simulink model "RL_Check"  (R2020a)
settings: Solver=FixedStepAuto  StartTime=0.0  StopTime=10.0  FixedStep=1e-4  RelTol=1e-3
libraries: commchan3 x1
settings Model: Creator=niranjan.bhujel  LastModifiedBy=niranjan.bhujel

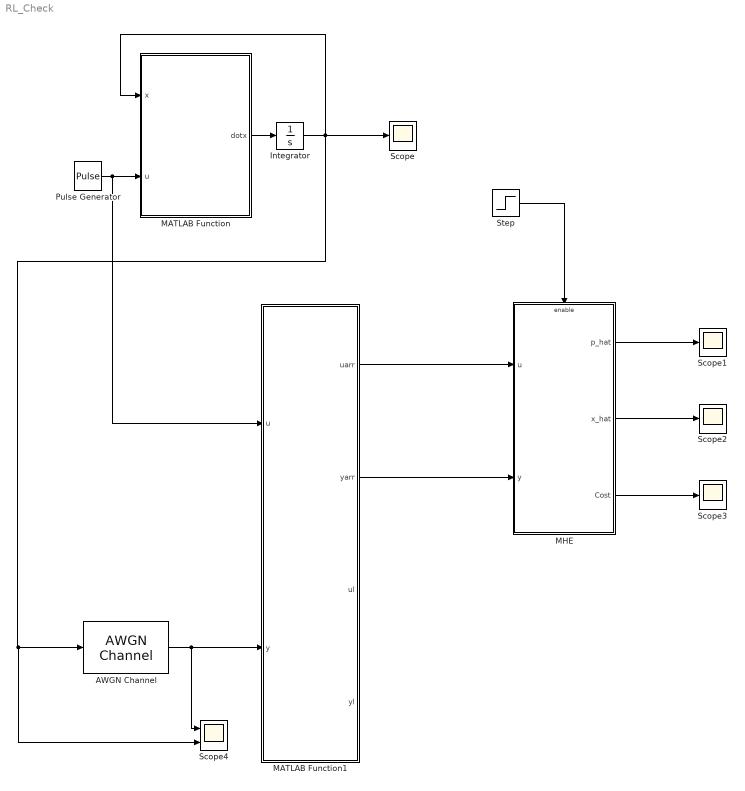
== system RL_Check ==
  AWGN Channel : commchan3/AWGN Channel  InputProcessing=Columns as channels (frame based)  seed=67  noiseMode=Variance from mask  EbNodB=10  EsNodB=10  SNRdB=10  bitsPerSym=1  Ps=1  Tsym=1  variance=1e-3
  Integrator : Integrator
  MATLAB Function : MATLAB Function  TreatAsAtomicUnit=on
  MATLAB Function1 : MATLAB Function  TreatAsAtomicUnit=on  SystemSampleTime=0.005
  MHE : Subsystem
  Pulse Generator : DiscretePulseGenerator  PulseType=Time based  Period=0.5  PulseWidth=50
  Scope{,1..3} (4 alike) : Scope
  Scope4 : Scope  NumInputPorts=2
  Step : Step  Time=5  SampleTime=0
  wires:
  MATLAB Function/1(dotx) -> Integrator/1
  Integrator/1 -> Scope4/2, AWGN Channel/1, Scope/1, MATLAB Function/1(x)
  Pulse Generator/1 -> MATLAB Function1/1(u), MATLAB Function/2(u)
  MATLAB Function1/1(uarr) -> MHE/1(u)
  MATLAB Function1/2(yarr) -> MHE/2(y)
  MHE/1(p_hat) -> Scope1/1
  MHE/2(x_hat) -> Scope2/1
  MHE/3(Cost) -> Scope3/1
  Step/1 -> MHE/Enable
  AWGN Channel/1 -> Scope4/1, MATLAB Function1/2(y)

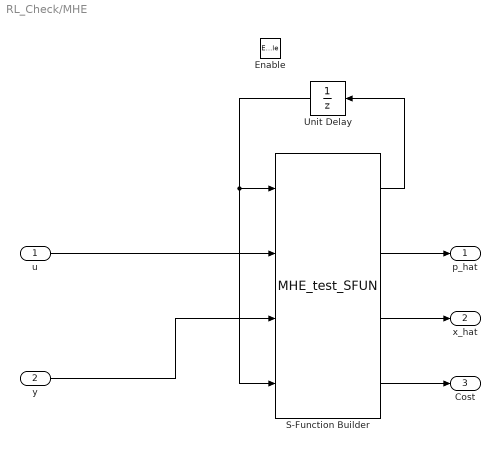
== system RL_Check/MHE ==
  u : Inport
  y : Inport  Port=2
  Enable : EnablePort
  S-Function Builder : S-Function  InitFcn=try, set_param(gcb,'FunctionName','MHE_test_SFUN'), end  FunctionName=MHE_test_SFUN  SFunctionModules=MHE_test_SFUN_wrapper MHE_Code MHE_Code_Call  SFunctionDeploymentMode=off  EnableBusSupport=off  mask(S-Function Builder){}
      mask help: Simulink:masks:SFunctionBuilder_MD
      mask init:
      | val = [[.9  0.75 0.75 1 1 .9 .9 1]',[1 1 0.75 0.75 .9 .9 1 .9]'];try , sys = get_param(gcb,'SfunBuilderFcnName');if isempty(sys), sys = get_param(gcb,'FunctionName'); end,catch, sys = get_param(gcb,'FunctionName'); end
      settings: CopyFcn=set_param(gcbh,'LinkStatus','none')  PreSaveFcn=try, set_param(gcb,'FunctionName','MHE_test_SFUN'), end  OpenFcn=sfunctionwizard(gcbh)
      mask Display: plot(val(:,1),val(:,2)),disp(sys), port_label('input',1,'zGuess'), port_label('input',2,'um'), port_label('input',3,'ym'), port_label('input',4,'zOp'), port_label('output',1,'zOut'), port_label('output',2,'p_hat'), port_label('output',3,'x_hat'), port_label('output',4,'Cost')
  Unit Delay : UnitDelay  InitialCondition=[0.1; zeros(13, 1)]  SampleTime=0.005  HasFrameUpgradeWarning=on
  p_hat : Outport
  x_hat : Outport  Port=2
  Cost : Outport  Port=3
  wires:
  S-Function Builder/1 -> Unit Delay/1
  S-Function Builder/3 -> x_hat/1
  S-Function Builder/4 -> Cost/1
  S-Function Builder/2 -> p_hat/1
  Unit Delay/1 -> S-Function Builder/4, S-Function Builder/1
  y/1 -> S-Function Builder/3
  u/1 -> S-Function Builder/2

== matlab function RL_Check/MATLAB Function1 ==
  data: u input; uarr output; y input; yarr output; ul output; yl output
function [uarr, yarr, ul, yl]= DataCollect(u, y)
    N=12;
    nu=1;
    ny=1;

    persistent x;
    if isempty(x)
        x = zeros(nu+ny, N+1);
    end

    ul = x(1:nu, 1);
    yl = x(nu+1:end, 1);

    for k=1:N
        x(:,k) = x(:,k+1);
    end
    x(:,N+1) = [u; y];

    uarr = x(1:nu, 1:N);
    yarr = x(nu+1:end,1:N+1);
end

== matlab function RL_Check/MATLAB Function ==
  data: x input; u input; dotx output
function dotx = fcn(x, u)
    R = 1;
    L = 0.1;
    
    dotx = -R/L*x + 1/L*u;
